simulink library "optimizeTrajectory_ul"  (R2022a)
settings: Solver=VariableStepAuto  StartTime=0.0  StopTime=10.0  RelTol=1e-3
values from neighbouring files (symbols this model uses):
  hiLvlCtrl = block.DialogPrm(2).Data    [optimizeAltitude_Lvl2SFun.m]    (also in optimizeThrLenghtAndElevation_Lvl2sFun.m; optimizeTrajectory_Lvl2SFun.m)
  mpckfgp = block.DialogPrm(1).Data    [optimizeAltitude_Lvl2SFun.m]    (also in optimizeAltitude_init.m = GP.KalmanFilteredGaussianProcess(hiLvlCtrl.spatialCovFn,    ; optimizeTrajectory_Lvl2SFun.m; optimizeTrajectory_init.m = GP.KalmanFilteredGaussianProcess(hiLvlCtrl.spatialCovFn,    )
settings Model: Creator=Ayaz  LastModifiedBy=lhill8
settings SolverCC: AlgebraicLoopSolver=TrustRegion
settings DebuggingCC: UnconnectedInputMsg=warning  UnconnectedOutputMsg=warning  UnconnectedLineMsg=warning  SFMachineParentedDataDiag=warning

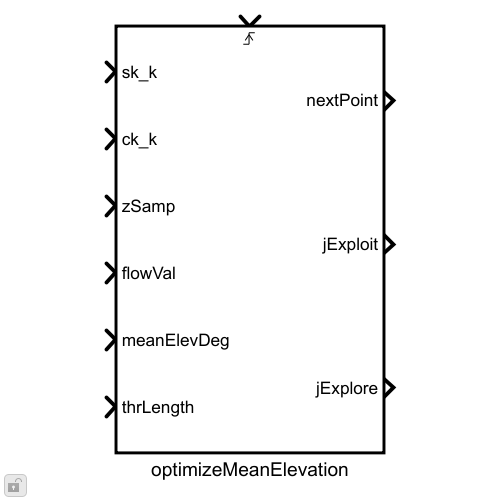
[thumbnail: Simulink's stored preview of the top-level diagram]
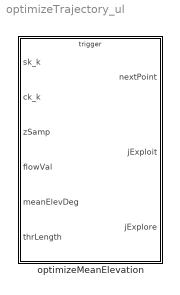
== system optimizeTrajectory_ul ==
  optimizeMeanElevation : Subsystem  mask{hiLvlCtrl=hiLvlCtrl}
      mask prompts: hiLvlCtrl "High level controller object"
      mask init:
      | optimizeTrajectory_init

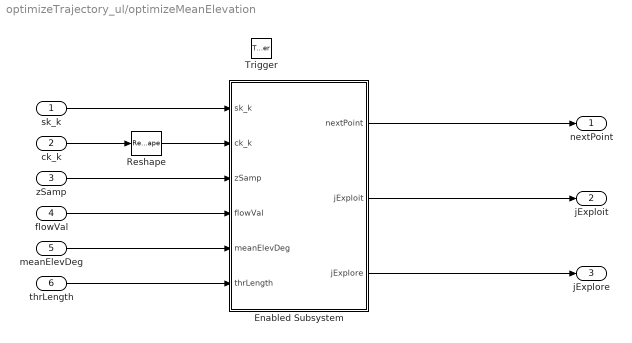
== system optimizeTrajectory_ul/optimizeMeanElevation ==
  sk_k : Inport
  ck_k : Inport  Port=2
  zSamp : Inport  Port=3
  flowVal : Inport  Port=4
  meanElevDeg : Inport  Port=5
  thrLength : Inport  Port=6
  Trigger : TriggerPort  VariantControl=Variant
  Enabled Subsystem : Subsystem  TreatAsAtomicUnit=on
  Reshape : Reshape  OutputDimensionality=Column vector (2-D)
  nextPoint : Outport
  jExploit : Outport  Port=2
  jExplore : Outport  Port=3
  wires:
  Enabled Subsystem/2(jExploit) -> jExploit/1
  Enabled Subsystem/3(jExplore) -> jExplore/1
  flowVal/1 -> Enabled Subsystem/4(flowVal)
  zSamp/1 -> Enabled Subsystem/3(zSamp)
  ck_k/1 -> Reshape/1
  sk_k/1 -> Enabled Subsystem/1(sk_k)
  meanElevDeg/1 -> Enabled Subsystem/5(meanElevDeg)
  thrLength/1 -> Enabled Subsystem/6(thrLength)
  Reshape/1 -> Enabled Subsystem/2(ck_k)
  Enabled Subsystem/1(nextPoint) -> nextPoint/1

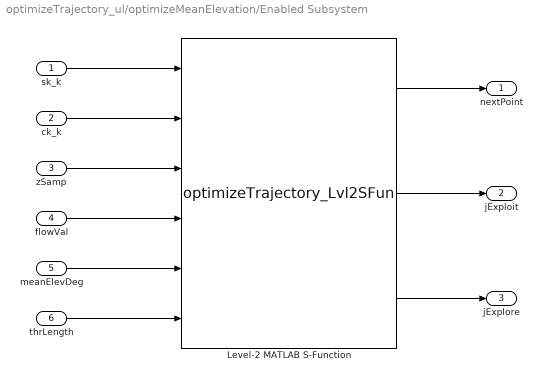
== system optimizeTrajectory_ul/optimizeMeanElevation/Enabled Subsystem ==
  sk_k : Inport
  ck_k : Inport  Port=2
  zSamp : Inport  Port=3
  flowVal : Inport  Port=4
  meanElevDeg : Inport  Port=5
  thrLength : Inport  Port=6
  Level-2 MATLAB S-Function : M-S-Function  FunctionName=optimizeTrajectory_Lvl2SFun  Parameters=mpckfgp,hiLvlCtrl
  nextPoint : Outport
  jExploit : Outport  Port=2
  jExplore : Outport  Port=3
  wires:
  meanElevDeg/1 -> Level-2 MATLAB S-Function/5
  thrLength/1 -> Level-2 MATLAB S-Function/6
  Level-2 MATLAB S-Function/1 -> nextPoint/1
  Level-2 MATLAB S-Function/2 -> jExploit/1
  Level-2 MATLAB S-Function/3 -> jExplore/1
  flowVal/1 -> Level-2 MATLAB S-Function/4
  zSamp/1 -> Level-2 MATLAB S-Function/3
  sk_k/1 -> Level-2 MATLAB S-Function/1
  ck_k/1 -> Level-2 MATLAB S-Function/2
